simulink model "lab05_KF_Blok"  (Simulink 9.0)
settings: Solver=FixedStepAuto  StartTime=0.0  StopTime=1.0  FixedStep=0.001  MaxStep=0.005  RelTol=1e-3  EnableMultiTasking=on
InitFcn:
  | % Parametry obiektu
  | R = 3;
  | L = 0.05;
  | kfi = 2.23;
  | J = 0.11;
  | 
  | global P
  | P = eye(2); % macierz kowariancji
settings Model: Creator=Jacek  LastModifiedBy=Jacek
settings DataIOCC: LimitDataPoints=on
settings DebuggingCC: UnderspecifiedInitializationDetection=Simplified  MergeDetectMultiDrivingBlocksExec=error  SolverPrmCheckMsg=warning
settings GRTTargetCC: GeneratePreprocessorConditionals=Disable all
settings ConfigComp: CovSFcnEnable=off

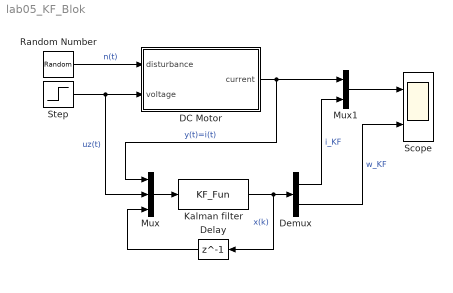
== system lab05_KF_Blok ==
  DC Motor : Subsystem
  Delay : Delay  DelayLength=1  InitialCondition=[0; 40]
  Demux : Demux  Outputs=2
  Kalman filter : MATLABFcn  MATLABFcn=KF_Fun
  Mux : Mux  Inputs=3
  Mux1 : Mux  Inputs=2
  Random Number : RandomNumber  Variance=10
  Scope : Scope  NumInputPorts=2
  Step : Step  Time=0  After=300  SampleTime=0
  wires:
  Random Number/1 -> DC Motor/1(disturbance)  "n(t)"
  Step/1 -> Mux/2, DC Motor/2(voltage)  "uz(t)"
  DC Motor/1(current) -> Mux/1, Mux1/1  "y(t)=i(t)"
  Mux1/1 -> Scope/1
  Demux/1 -> Mux1/2  "i_KF"
  Demux/2 -> Scope/2  "w_KF"
  Kalman filter/1 -> Delay/1, Demux/1  "x(k)"
  Delay/1 -> Mux/3
  Mux/1 -> Kalman filter/1

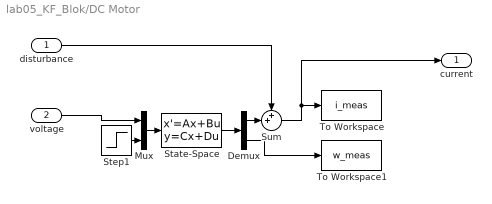
== system lab05_KF_Blok/DC Motor ==
  disturbance : Inport
  voltage : Inport  Port=2
  Demux : Demux  Outputs=2
  Mux : Mux  Inputs=2
  State-Space : StateSpace  A=[-3/0.05, -2.23/0.05; 2.23/0.11, 0]  B=[1/0.05 0; 0 -1/0.11]  C=[1 0;0 1]  D=[0 0; 0 0]  InitialCondition=[0 ;40]
  Step1 : Step  Time=0.5  After=44.6  SampleTime=0
  Sum : Sum  Inputs=++|
  To Workspace : ToWorkspace  VariableName=i_meas  SampleTime=-1
  To Workspace1 : ToWorkspace  VariableName=w_meas  SampleTime=-1
  current : Outport
  wires:
  Mux/1 -> State-Space/1
  voltage/1 -> Mux/1
  Step1/1 -> Mux/2
  State-Space/1 -> Demux/1
  Sum/1 -> current/1, To Workspace/1
  Demux/1 -> Sum/2
  disturbance/1 -> Sum/1
  Demux/2 -> To Workspace1/1
